simulink model "benzetim"  (R2022b)
settings: Solver=VariableStepAuto  StartTime=0.0  StopTime=10.0  RelTol=1e-3
libraries: simulink_extras x3
settings Model: Creator=Nikola  LastModifiedBy=Nikola

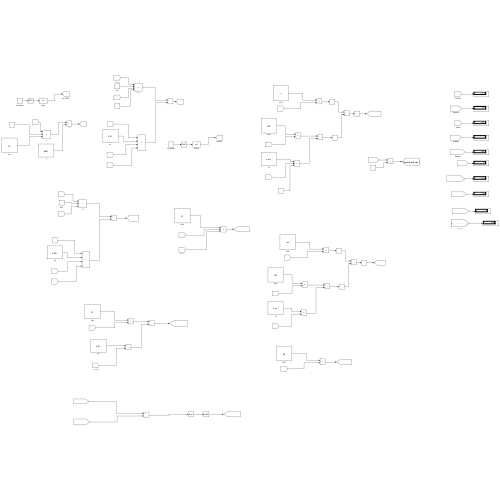
[thumbnail: Simulink's stored preview of the top-level diagram]
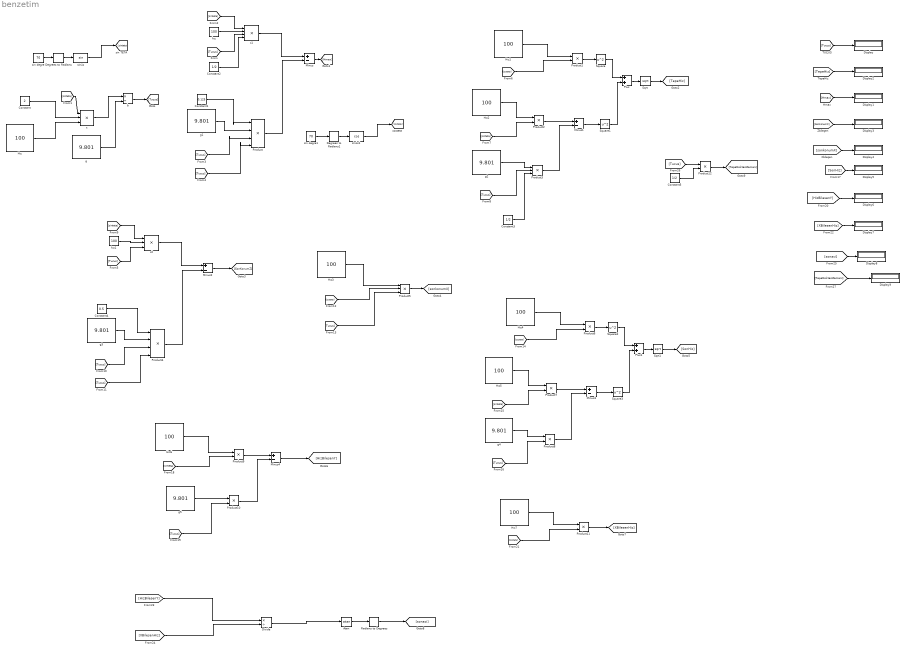
== system benzetim ==
  Atan : Trigonometry  Operator=atan
  Constant : Constant  Value=2
  Constant1 : Constant  Value=0.125
  Constant2 : Constant  Value=1/2
  Constant3 : Constant  Value=1/2
  Constant4 : Constant  Value=0.5
  Constant5 : Constant  Value=1/2
  Degrees to Radians : simulink_extras/Transformations/Degrees to Radians
  Degrees to Radians1 : simulink_extras/Transformations/Degrees to Radians
  Display{,1..9} (10 alike) : Display
  Divide : Product  Inputs=*/
  Hız{,1..7} (8 alike) : Constant  Value=100
  Minus{,1..4} (5 alike) : Sum  Inputs=+-
  Plus : Sum
  Plus1 : Sum
  Product : Product  Inputs=4
  Product{1..2,6..12} (9 alike) : Product
  Product3 : Product  Inputs=3
  Product4 : Product  Inputs=4
  Product5 : Product  Inputs=3
  Radians to Degrees : simulink_extras/Transformations/Radians to Degrees
  Sqrt : Sqrt
  Sqrt1 : Sqrt
  Square{,1..3} (4 alike) : Math  Operator=square  SignedPower=on  RndMeth=Zero
  b : Product  Inputs=*/
  c : Product  Inputs=3
  c1 : Product  Inputs=4
  c2 : Product  Inputs=3
  g{,1..5} (6 alike) : Constant  Value=9.801
  hız : Constant  Value=100
  hız1 : Constant  Value=100
  sin degre : Constant  Value=70
  sin degre1 : Constant  Value=70
  sinüs : Trigonometry
  sinüs1 : Trigonometry  Operator=cos
  wires:
  sin degre/1 -> Degrees to Radians/1
  Degrees to Radians/1 -> sinüs/1
  Hız/1 -> c/3
  Constant/1 -> c/2
  c/1 -> b/1
  g/1 -> b/2
  b/1 -> [Tucus]
  sinüs/1 -> [sinteta]
  [sinteta] -> c/1
  hız/1 -> c1/2
  [sinteta] -> c1/1
  [Tucus] -> c1/3
  [Tucus] -> Display/1
  c1/1 -> Minus/1
  Constant1/1 -> Product/1
  g1/1 -> Product/2
  [Tucus] -> Product/3
  [Tucus] -> Product/4
  Product/1 -> Minus/2
  Minus/1 -> [Hmax]
  [Hmax] -> Display1/1
  Constant2/1 -> c1/4
  sinüs1/1 -> [costeta]
  Degrees to Radians1/1 -> sinüs1/1
  sin degre1/1 -> Degrees to Radians1/1
  Hız1/1 -> Product1/1
  [costeta] -> Product1/2
  Product1/1 -> Square/1
  Square/1 -> Plus/1
  [sinteta] -> Product2/2
  Hız2/1 -> Product2/1
  Product2/1 -> Minus1/1
  g2/1 -> Product3/1
  [Tucus] -> Product3/2
  Constant3/1 -> Product3/3
  Product3/1 -> Minus1/2
  Minus1/1 -> Square1/1
  Square1/1 -> Plus/2
  Plus/1 -> Sqrt/1
  [TepeHiz] -> Display2/1
  Sqrt/1 -> [TepeHiz]
  [sinteta] -> c2/1
  c2/1 -> Minus2/1
  [Tucus] -> c2/3
  Product4/1 -> Minus2/2
  g3/1 -> Product4/2
  hız1/1 -> c2/2
  Minus2/1 -> [SonKonumZ]
  [SonKonumZ] -> Display3/1
  [Tucus] -> Product4/4
  [Tucus] -> Product4/3
  Constant4/1 -> Product4/1
  [Tucus] -> Product5/3
  [costeta] -> Product5/2
  Hız3/1 -> Product5/1
  Product5/1 -> [sonkonumX]
  [sonkonumX] -> Display4/1
  [sinteta] -> Product7/2
  Minus3/1 -> Square3/1
  Product6/1 -> Square2/1
  [Tucus] -> Product8/2
  [costeta] -> Product6/2
  Product7/1 -> Minus3/1
  Square2/1 -> Plus1/1
  Square3/1 -> Plus1/2
  Sqrt1/1 -> [SonHiz]
  Hız5/1 -> Product7/1
  g4/1 -> Product8/1
  Product8/1 -> Minus3/2
  Hız4/1 -> Product6/1
  Plus1/1 -> Sqrt1/1
  [SonHiz] -> Display5/1
  Hız6/1 -> Product9/1
  [sinteta] -> Product9/2
  Product9/1 -> Minus4/1
  g5/1 -> Product10/1
  [Tucus] -> Product10/2
  Product10/1 -> Minus4/2
  Minus4/1 -> [HizBilesenY]
  [HizBilesenY] -> Display6/1
  Product11/1 -> [XBilesenHiz]
  Hız7/1 -> Product11/1
  [costeta] -> Product11/2
  [XBilesenHiz] -> Display7/1
  [HizBilesenY] -> Divide/1
  [XBilesenHiz] -> Divide/2
  Divide/1 -> Atan/1
  Atan/1 -> Radians to Degrees/1
  Radians to Degrees/1 -> [sonaci]
  [sonaci] -> Display8/1
  [Tucus] -> Product12/1
  Constant5/1 -> Product12/2
  Product12/1 -> [TepeNoktasiZamani]
  [TepeNoktasiZamani] -> Display9/1
